simulink model "PROJEKAT3_EKSPERIMENTALNA_SHEMA"  (R2015b)
settings: Solver=ode3  StartTime=0.0  StopTime=inf  FixedStep=0.001  RelTol=1e-3
undefined symbols (not defined in the file): analoginput, analogoutput
libraries: daqlib x2, simulink x2
settings Model: Creator=Lab-Administrator  LastModifiedBy=Avdo1
settings DataIOCC: SaveFormat=Array
settings DebuggingCC: UnderspecifiedInitializationDetection=Classic  MergeDetectMultiDrivingBlocksExec=none  SolverPrmCheckMsg=warning  StateNameClashWarn=warning
settings HardwareCC: ProdBitPerPointer=32  ProdLargestAtomicFloat=None  ProdIntDivRoundTo=Undefined  ProdEndianess=Unspecified  ProdWordSize=32  ProdHWDeviceType=32-bit Generic
settings GRTTargetCC: GeneratePreprocessorConditionals=Disable all
settings ConfigComp: CovModelRefEnable=Off

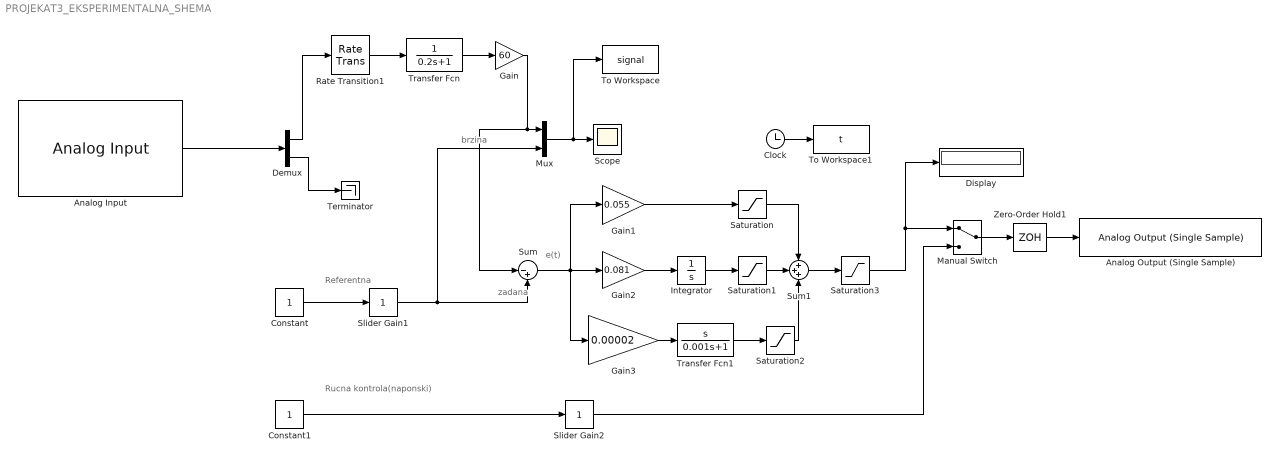
== system PROJEKAT3_EKSPERIMENTALNA_SHEMA ==
  note: Referentna
  note: Rucna kontrola(naponski)
  note: zadana
  note: brzina
  note: e(t)
  Analog Input : daqlib/Analog Input  AcqMode=0  DeviceMenu=winsound 0 (Microphone (Realtek(R) Audio))  Device=nidaq Dev1 (PCI-6024E)  ObjConstructor=analoginput('nidaq','Dev1')  SampleRate=1000  ActualRate=1000  SamplesPerFrame=2  InputType=SingleEnded  NChannelsSelected=1  Channels=0$0$$1$#0$1$$1$#0$2$$1$#1$3$$1$#0$4$$1$#0$5$$1$#0$6$$1$#0$7$$1$#0$8$$1$#0$9$$1$#0$10$$1$#0$11$$1$#0$12$$1$#0$13$$1$#0$14$$1$#0$15$$1$#  NPorts=1 per hardware channel  DataType=double
      settings: SignalType=Sample-based
  Analog Output (Single Sample) : daqlib/Analog Output (Single Sample)  DeviceMenu=winsound 0 (Microphone (Realtek(R) Audio))  Device=nidaq Dev1 (PCI-6024E)  ObjConstructor=analogoutput('nidaq','Dev1')  NChannelsSelected=1  Channels=1$0$$1$0$#0$1$$1$0$#  NPorts=1 per hardware channel
  Clock : Clock
  Constant : Constant
  Constant1 : Constant
  Demux : Demux  Outputs=2
  Display : Display
  Gain : Gain  Gain=60
  Gain1 : Gain  Gain=0.055
  Gain2 : Gain  Gain=0.081
  Gain3 : Gain  Gain=0.00002
  Integrator : Integrator  LimitOutput=on  UpperSaturationLimit=10  LowerSaturationLimit=-10
  Manual Switch : ManualSwitch
  Mux : Mux  Inputs=2
  Rate Transition1 : RateTransition
  Saturation{,1..3} (4 alike) : Saturate  UpperLimit=10  LowerLimit=0
  Scope : Scope
  Slider Gain1 : simulink/Math Operations/Slider Gain  low=0  gain=1  high=2
  Slider Gain2 : simulink/Math Operations/Slider Gain  low=0  gain=1  high=2
  Sum : Sum  Inputs=|-+
  Sum1 : Sum  Inputs=+++
  Terminator : Terminator
  To Workspace : ToWorkspace  VariableName=signal  SampleTime=0.001
  To Workspace1 : ToWorkspace  VariableName=t  SampleTime=0.001
  Transfer Fcn : TransferFcn  Denominator=[0.2 1]
  Transfer Fcn1 : TransferFcn  Numerator=[1 0]  Denominator=[0.001 1]
  Zero-Order Hold1 : ZeroOrderHold  SampleTime=0.001
  wires:
  Demux/2 -> Terminator/1
  Clock/1 -> To Workspace1/1
  Analog Input/1 -> Demux/1
  Gain/1 -> Sum/1, Mux/1
  Transfer Fcn/1 -> Gain/1
  Constant/1 -> Slider Gain1/1
  Mux/1 -> To Workspace/1, Scope/1
  Constant1/1 -> Slider Gain2/1
  Gain1/1 -> Saturation/1
  Saturation/1 -> Sum1/1
  Saturation1/1 -> Sum1/2
  Saturation2/1 -> Sum1/3
  Sum1/1 -> Saturation3/1
  Gain2/1 -> Integrator/1
  Integrator/1 -> Saturation1/1
  Saturation3/1 -> Display/1, Manual Switch/1
  Sum/1 -> Gain3/1, Gain2/1, Gain1/1
  Demux/1 -> Rate Transition1/1
  Rate Transition1/1 -> Transfer Fcn/1
  Gain3/1 -> Transfer Fcn1/1
  Manual Switch/1 -> Zero-Order Hold1/1
  Zero-Order Hold1/1 -> Analog Output (Single Sample)/1
  Slider Gain1/1 -> Sum/2, Mux/2
  Slider Gain2/1 -> Manual Switch/2
  Transfer Fcn1/1 -> Saturation2/1
